simulink model "s2"  (Simulink 2.00)
settings: Solver=ode15s  StartTime=0.0  StopTime=tstop  MaxStep=0.0010  RelTol=1e-5  AbsTol=1e-6
values from neighbouring files (symbols this model uses):
  C = 1000e-6    (= 0.001)    [M2.M]    (also in M2INIT.M; M4.M = 1.082251e-07)
  iLo = 0    [M2.M]    (also in M2INIT.M; M3.M; M4.M)
  L = 0.1    [M2.M]    (also in M2INIT.M; M3.M = 0.04; M4.M = 0.000231)
  Rs = 50    [M2.M]    (also in M2INIT.M)
  tdelay = 0.05    [M2.M]    (also in M2INIT.M)
  vCo = 0    [M2.M]    (also in M2INIT.M; M4.M)
  VS_mag = 100    [M2.M]    (also in M2INIT.M)
settings Model: SaveTime=off  SaveOutput=off  ConsistencyChecking=off

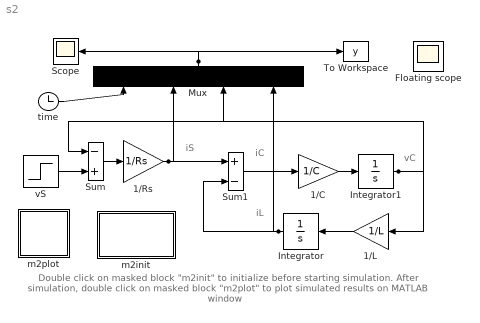
== system s2 ==
  note: vC
  note: iL
  note: iC
  note: iS
  note: Double click on masked block "m2init" to initialize before starting
      | simulation. After simulation, double click on masked block "m2plot"
      | to plot simulated results on MATLAB window
  1/C : Gain  Gain=1/C
  1/L : Gain  Orientation=left  Gain=1/L
  1/Rs : Gain  Gain=1/Rs
  m2init : Subsystem
      settings: OpenFcn=m2init
      mask Type: Masked block of m2init.m
      mask Help: Uses m2init.m to initialize
      mask Display: disp('Initialize\nm2SIM')
  m2plot : Subsystem
      settings: OpenFcn=m2plot
      mask Type: Masked block of m2plot.m
      mask Help: Uses m2plot.m to plot
      mask Display: disp('Plot\nresults')
  Floating scope : Scope
      settings: Floating=on  TickLabels=on  TimeRange=auto  YMin=-5  YMax=5  SaveToWorkspace=off  SaveName=ScopeData  LimitMaxRows=off
  Integrator : Integrator  Orientation=left  ExternalReset=none  InitialConditionSource=internal  InitialCondition=iLo  LimitOutput=off  UpperSaturationLimit=inf  LowerSaturationLimit=-inf  ShowSaturationPort=off  ShowStatePort=off  AbsoluteTolerance=auto
  Integrator1 : Integrator  ExternalReset=none  InitialConditionSource=internal  InitialCondition=vCo  LimitOutput=off  UpperSaturationLimit=inf  LowerSaturationLimit=-inf  ShowSaturationPort=off  ShowStatePort=off  AbsoluteTolerance=auto
  Mux : Mux  Orientation=up  Inputs=4
  Scope : Scope
      settings: TickLabels=on  TimeRange=auto  YMin=-5  YMax=5  SaveToWorkspace=off  SaveName=ScopeData
  Sum : Sum  Inputs=-+
  Sum1 : Sum  Inputs=+-
  To Workspace : ToWorkspace  VariableName=y  SampleTime=0
      settings: Buffer=3000
  time : Clock
      settings: DeleteFcn=simclock BlockIsBeingDestroyed  PostSaveFcn=simclock Save
  vS : Step  Time=tdelay  Before=0  After=VS_mag
  wires:
  Sum/1 -> 1/Rs/1
  Sum1/1 -> 1/C/1
  1/C/1 -> Integrator1/1
  1/L/1 -> Integrator/1
  time/1 -> Mux/1
  Mux/1 -> To Workspace/1, Scope/1
  vS/1 -> Sum/2
  1/Rs/1 -> Sum1/1, Mux/2
  Integrator/1 -> Sum1/2, Mux/4
  Integrator1/1 -> Sum/1, Mux/3, 1/L/1

== system s2/m2init ==
  note: Initialize above simulation
      | using the values given in
      | m2init.

== system s2/m2plot ==
  note: Display the plots programmed in
      | m2plot.m in a new figure window
